simulink model "pitch_loop"  (R2019a)
settings: Solver=VariableStepAuto  StartTime=0.0  StopTime=10000  RelTol=1e-3
undefined symbols (not defined in the file or in its folder): AP, trans_func
settings Model: Creator=nikhil  LastModifiedBy=VTOL_HYD

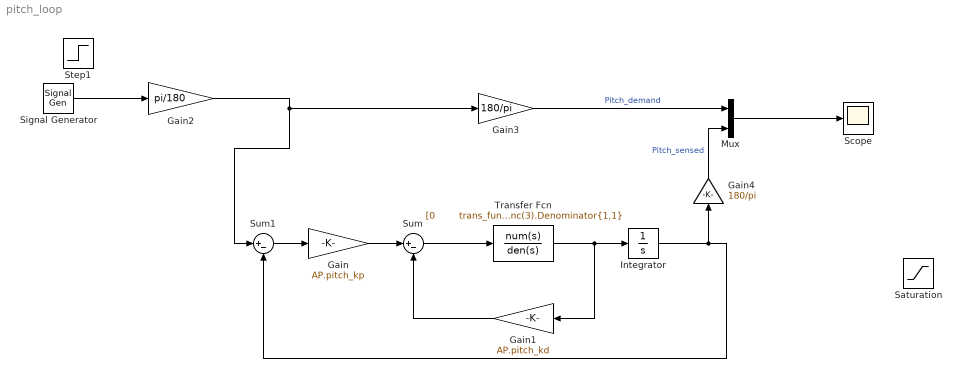
== system pitch_loop ==
  Gain : Gain  Gain=AP.pitch_kp
  Gain1 : Gain  Gain=AP.pitch_kd
  Gain2 : Gain  Gain=pi/180
  Gain3 : Gain  Gain=180/pi
  Gain4 : Gain  Gain=180/pi
  Integrator : Integrator
  Mux : Mux  Inputs=2
  Saturation : Saturate  UpperLimit=3.14  LowerLimit=-3.14
  Scope : Scope
  Signal Generator : SignalGenerator  Amplitude=25  Frequency=.01  Units=rad/sec
  Step1 : Step  Time=8  After=45  SampleTime=5
  Sum : Sum  Inputs=|+-
  Sum1 : Sum  Inputs=|+-
  Transfer Fcn : TransferFcn  Numerator="[0        trans_func(3).Numerator{1,1}(3)       0]"  Denominator=trans_func(3).Denominator{1,1}
  wires:
  Sum/1 -> Transfer Fcn/1
  Gain/1 -> Sum/1
  Sum1/1 -> Gain/1
  Gain2/1 -> Sum1/1, Gain3/1
  Mux/1 -> Scope/1
  Transfer Fcn/1 -> Gain1/1, Integrator/1
  Gain1/1 -> Sum/2
  Gain3/1 -> Mux/1  "Pitch_demand"
  Integrator/1 -> Gain4/1, Sum1/2
  Gain4/1 -> Mux/2  "Pitch_sensed"
  Signal Generator/1 -> Gain2/1
